simulink model "INS"  (R2018b)
settings: configuration reference "ins_config" (kept outside this file)
values from neighbouring files (symbols this model uses):
  INS_EXPORT = Simulink.Parameter(INS_EXPORT_VALUE)    [ins_model_init.m]
  INS_PARAM = Simulink.Parameter(INS_PARAM_VALUE)    [ins_model_init.m]
undefined symbols (not defined in the file or in its folder): DiscIntNeverNeededParam, INS_CONST, INS_EXPORT_VALUE
libraries: simulink x90, FMT_Model_Lib x31
(part 3 of 4)

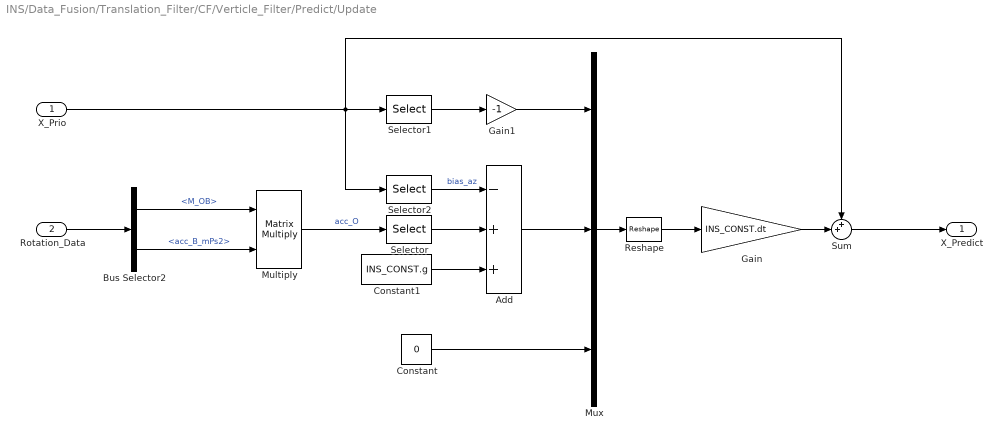
== system INS/Data_Fusion/Translation_Filter/CF/Verticle_Filter/Predict/Update ==
  X_Prio : Inport
  Rotation_Data : Inport  Port=2
  Add : Sum  Inputs=-++
  Bus Selector2 : BusSelector  OutputSignals=M_OB,acc_B_mPs2
  Constant : Constant  Value=0  OutDataTypeStr=single
  Constant1 : Constant  Value=INS_CONST.g  OutDataTypeStr=single
  Gain : Gain  Gain=INS_CONST.dt  OutDataTypeStr=Inherit: Same as input
  Gain1 : Gain  Gain=-1  OutDataTypeStr=Inherit: Same as input
  Multiply : Product  Multiplication=Matrix(*)
  Mux : Mux  Inputs=3
  Reshape : Reshape  OutputDimensionality=Customize  OutputDimensions=[3,1]
  Selector : Selector  InputPortWidth=3  IndexOptions=Index vector (dialog)  Indices=[3]  OutputSizes=1
  Selector1 : Selector  InputPortWidth=3  IndexOptions=Index vector (dialog)  Indices=[2]  OutputSizes=1
  Selector2 : Selector  InputPortWidth=3  IndexOptions=Index vector (dialog)  Indices=[3]  OutputSizes=1
  Sum : Sum  Inputs=++|
  X_Predict : Outport
  wires:
  Rotation_Data/1 -> Bus Selector2/1
  Bus Selector2/1 -> Multiply/1  "<M_OB>"
  Multiply/1 -> Selector/1  "acc_O"
  Bus Selector2/2 -> Multiply/2  "<acc_B_mPs2>"
  X_Prio/1 -> Selector2/1, Sum/1, Selector1/1
  Selector1/1 -> Gain1/1
  Constant/1 -> Mux/3
  Mux/1 -> Reshape/1
  Reshape/1 -> Gain/1
  Sum/1 -> X_Predict/1
  Add/1 -> Mux/2
  Constant1/1 -> Add/3
  Selector2/1 -> Add/1  "bias_az"
  Gain1/1 -> Mux/1
  Gain/1 -> Sum/2
  Selector/1 -> Add/2

== system INS/Data_Fusion/Translation_Filter/TF_Data_PreProcess/Sensor_Process/Sensor_Select/Horizontal_Sensor_Select ==
  Sensor_Status : Inport
  Bus Creator : BusCreator  Inputs=1
  Bus Selector : BusSelector  OutputSignals=GPS_Status.gps_vaid,GPS_Status.spd_valid,GPS_Status.pos_valid
  Compare To Zero2 : simulink/Logic and Bit Operations/Compare To Zero  relop=>  OutDataTypeStr=boolean
  Logical Operator : Logic  Inputs=3  AllPortsSameDT=off  OutDataTypeStr=boolean
  Min : MinMax
  horizon_select : Outport
  wires:
  Bus Selector/1 -> Logical Operator/1  "<gps_vaid>"
  Logical Operator/1 -> Min/1
  Min/1 -> Compare To Zero2/1
  Compare To Zero2/1 -> Bus Creator/1  "gps_enable"
  Sensor_Status/1 -> Bus Selector/1
  Bus Creator/1 -> horizon_select/1
  Bus Selector/2 -> Logical Operator/2  "<spd_valid>"
  Bus Selector/3 -> Logical Operator/3  "<pos_valid>"

== system INS/Data_Fusion/Translation_Filter/TF_Data_PreProcess/Sensor_Process/Sensor_Select/Vertical_Sensor_Select ==
  Sensor_Status : Inport
  Bus Creator : BusCreator  Inputs=2
  Bus Selector : BusSelector  OutputSignals=GPS_Status.gps_vaid,GPS_Status.spd_valid,GPS_Status.alt_valid
  Bus Selector2 : BusSelector  OutputSignals=Baro_Status.baro_valid
  Compare To Zero1 : simulink/Logic and Bit Operations/Compare To Zero  relop=>  OutDataTypeStr=boolean
  Compare To Zero4 : simulink/Logic and Bit Operations/Compare To Zero  relop=>  OutDataTypeStr=boolean
  Compare To Zero6 : simulink/Logic and Bit Operations/Compare To Zero  relop=>  OutDataTypeStr=boolean
  Data Type Conversion : DataTypeConversion  OutDataTypeStr=int8
  Data Type Conversion1 : DataTypeConversion  OutDataTypeStr=int8
  Logical Operator : Logic  Inputs=3  AllPortsSameDT=off  OutDataTypeStr=boolean
  Saturation : Saturate  UpperLimit=1  LowerLimit=0
  Saturation1 : Saturate  UpperLimit=1  LowerLimit=0
  Subtract : Sum  Inputs=-+
  vert_select : Outport
  wires:
  Data Type Conversion/1 -> Saturation/1
  Logical Operator/1 -> Data Type Conversion/1
  Saturation/1 -> Compare To Zero4/1, Subtract/1
  Bus Selector/2 -> Logical Operator/2  "<spd_valid>"
  Bus Selector2/1 -> Compare To Zero1/1  "<baro_valid>"
  Compare To Zero1/1 -> Data Type Conversion1/1
  Subtract/1 -> Saturation1/1
  Saturation1/1 -> Compare To Zero6/1
  Data Type Conversion1/1 -> Subtract/2
  Bus Selector/1 -> Logical Operator/1  "<gps_vaid>"
  Bus Selector/3 -> Logical Operator/3  "<alt_valid>"
  Compare To Zero4/1 -> Bus Creator/1  "gps_enable"
  Compare To Zero6/1 -> Bus Creator/2  "baro_enable"
  Sensor_Status/1 -> Bus Selector2/1, Bus Selector/1
  Bus Creator/1 -> vert_select/1

== system INS/Data_Fusion/Translation_Filter/TF_Data_PreProcess/Sensor_Process/TF_Sensor_Measures/Barometer_Meas ==
  Sensor_Data : Inport
  Bus Creator : BusCreator  Inputs=2
  Bus Selector1 : BusSelector  OutputSignals=Baro_Data.timestamp,Baro_Data.h_R_m
  Signal Copy1 : SignalConversion  OverrideOpt=off
  Signal Copy3 : SignalConversion  OverrideOpt=off
  Baro_Meas : Outport
  wires:
  Sensor_Data/1 -> Bus Selector1/1
  Bus Selector1/2 -> Signal Copy1/1  "<h_R_m>"
  Bus Creator/1 -> Baro_Meas/1
  Bus Selector1/1 -> Signal Copy3/1  "<timestamp>"
  Signal Copy3/1 -> Bus Creator/1  "timestamp_ms"
  Signal Copy1/1 -> Bus Creator/2  "h_R_m"

== system INS/Data_Fusion/Translation_Filter/TF_Data_PreProcess/Sensor_Process/TF_Sensor_Measures/GPS_Meas ==
  Sensor_Data : Inport
  Bus Creator : BusCreator  Inputs=12
  Bus Selector : BusSelector  OutputSignals=GPS_Data.dx_dlat,GPS_Data.dy_dlon,GPS_Data.dz_dh,GPS_Data.lat_rad,GPS_Data.lon_rad,GPS_Data.height_m,GPS_Data.vn_mPs,GPS_Data.ve_mPs,GPS_Data.vd_mPs,GPS_Data.timestamp_ms,GPS_Data.spd_quality,GPS_Data.pos_quality
  Signal Copy{,1..11} (12 alike) : SignalConversion  OverrideOpt=off
  GPS_Meas : Outport
  wires:
  Bus Selector/11 -> Signal Copy10/1  "<spd_quality>"
  Signal Copy9/1 -> Bus Creator/10  "timestamp_ms"
  Signal Copy8/1 -> Bus Creator/9  "vd_mPs"
  Signal Copy7/1 -> Bus Creator/8  "ve_mPs"
  Signal Copy6/1 -> Bus Creator/7  "vn_mPs"
  Signal Copy5/1 -> Bus Creator/6  "h_m"
  Signal Copy4/1 -> Bus Creator/5  "lon_rad"
  Signal Copy3/1 -> Bus Creator/4  "lat_rad"
  Signal Copy2/1 -> Bus Creator/3  "dz_dh"
  Signal Copy1/1 -> Bus Creator/2  "dy_dlon"
  Signal Copy/1 -> Bus Creator/1  "dx_dlat"
  Bus Selector/10 -> Signal Copy9/1  "<timestamp_ms>"
  Bus Selector/9 -> Signal Copy8/1  "<vd_mPs>"
  Bus Selector/8 -> Signal Copy7/1  "<ve_mPs>"
  Bus Selector/7 -> Signal Copy6/1  "<vn_mPs>"
  Bus Selector/6 -> Signal Copy5/1  "<height_m>"
  Bus Selector/5 -> Signal Copy4/1  "<lon_rad>"
  Bus Selector/4 -> Signal Copy3/1  "<lat_rad>"
  Bus Selector/3 -> Signal Copy2/1  "<dz_dh>"
  Bus Selector/2 -> Signal Copy1/1  "<dy_dlon>"
  Bus Selector/1 -> Signal Copy/1  "<dx_dlat>"
  Bus Creator/1 -> GPS_Meas/1
  Sensor_Data/1 -> Bus Selector/1
  Bus Selector/12 -> Signal Copy11/1  "<pos_quality>"
  Signal Copy10/1 -> Bus Creator/11  "spd_quality"
  Signal Copy11/1 -> Bus Creator/12  "pos_quality"

== system INS/Data_Fusion/Translation_Filter/TF_Data_PreProcess/Sensor_Process/TF_Sensor_Status/Barometer_Status ==
  Sensor_Data : Inport
  Bus Creator : BusCreator  Inputs=1
  Bus Selector : BusSelector  OutputSignals=Baro_Data.baro_valid
  Signal Copy : SignalConversion  OverrideOpt=off
  Baro_Status : Outport
  wires:
  Bus Selector/1 -> Signal Copy/1  "<baro_valid>"
  Bus Creator/1 -> Baro_Status/1
  Sensor_Data/1 -> Bus Selector/1
  Signal Copy/1 -> Bus Creator/1  "baro_valid"

== system INS/Data_Fusion/Translation_Filter/TF_Data_PreProcess/Sensor_Process/TF_Sensor_Status/GPS_Status ==
  Sensor_Data : Inport
  Bus Creator : BusCreator  Inputs=4
  Bus Selector : BusSelector  OutputSignals=GPS_Data.GPS_valid,GPS_Data.spd_quality,GPS_Data.pos_quality,GPS_Data.alt_quality
  Relay : Relay  OnSwitchValue=0.7  OffSwitchValue=0.3
  Relay1 : Relay  OnSwitchValue=0.7  OffSwitchValue=0.3
  Relay2 : Relay  OnSwitchValue=0.7  OffSwitchValue=0.3
  Signal Copy : SignalConversion  OverrideOpt=off
  GPS_Status : Outport
  wires:
  Bus Creator/1 -> GPS_Status/1
  Relay1/1 -> Bus Creator/3  "pos_valid"
  Relay/1 -> Bus Creator/2  "spd_valid"
  Signal Copy/1 -> Bus Creator/1  "gps_vaid"
  Bus Selector/3 -> Relay1/1  "<pos_quality>"
  Bus Selector/2 -> Relay/1  "<spd_quality>"
  Bus Selector/1 -> Signal Copy/1  "<GPS_valid>"
  Sensor_Data/1 -> Bus Selector/1
  Bus Selector/4 -> Relay2/1  "<alt_quality>"
  Relay2/1 -> Bus Creator/4  "alt_valid"

== system INS/Data_Fusion/Translation_Filter/TF_Data_PreProcess/Transfer_Filter_Control/Position_Reference/Bus_Constructor ==
  WGS84_pos_ref : Inport
  WGS84_dpos_ref : Inport  Port=2
  WGS84_hgt_ref : Inport  Port=3
  WGS84_dhgt_ref : Inport  Port=4
  Bus Creator : BusCreator  Inputs=2
  Bus Creator1 : BusCreator  Inputs=3
  Bus Creator2 : BusCreator  Inputs=3
  Demux : Demux  Outputs=2
  Demux1 : Demux  Outputs=2
  WGS84_Ref : Outport
  wires:
  Bus Creator/1 -> WGS84_Ref/1
  Demux/1 -> Bus Creator1/1  "dx_dlat_0"
  Demux1/1 -> Bus Creator2/1  "lat_0_rad"
  Demux/2 -> Bus Creator1/2  "dy_dlon_0"
  Demux1/2 -> Bus Creator2/2  "lon_0_rad"
  Bus Creator2/1 -> Bus Creator/2  "WGS84_pos_ref"
  WGS84_dhgt_ref/1 -> Bus Creator1/3  "dz_dh_0"
  WGS84_hgt_ref/1 -> Bus Creator2/3  "h_0_m"
  Bus Creator1/1 -> Bus Creator/1  "WGS84_derivatives_ref"
  WGS84_dpos_ref/1 -> Demux/1
  WGS84_pos_ref/1 -> Demux1/1

== system INS/Data_Fusion/Translation_Filter/TF_Data_PreProcess/Transfer_Filter_Control/Position_Reference/Bus_Select ==
  Sensor_Meas : Inport
  Bus Selector1 : BusSelector  OutputSignals=GPS_Meas.dx_dlat,GPS_Meas.dy_dlon,GPS_Meas.dz_dh,GPS_Meas.lat_rad,GPS_Meas.lon_rad,GPS_Meas.h_m
  Mux : Mux  Inputs=3
  Mux1 : Mux  Inputs=3
  WGS84_derivatives : Outport
  WGS84_position : Outport  Port=2
  wires:
  Mux1/1 -> WGS84_position/1
  Sensor_Meas/1 -> Bus Selector1/1
  Mux/1 -> WGS84_derivatives/1
  Bus Selector1/6 -> Mux1/3  "<h_m>"
  Bus Selector1/5 -> Mux1/2  "<lon_rad>"
  Bus Selector1/4 -> Mux1/1  "<lat_rad>"
  Bus Selector1/3 -> Mux/3  "<dz_dh>"
  Bus Selector1/2 -> Mux/2  "<dy_dlon>"
  Bus Selector1/1 -> Mux/1  "<dx_dlat>"

== system INS/Data_Fusion/Translation_Filter/TF_Data_PreProcess/Transfer_Filter_Control/Position_Reference/Height_Ref ==
  Translation_Data : Inport
  Sensor_Valid : Inport  Port=2
  WGS84_derivatives : Inport  Port=3
  WGS84_position : Inport  Port=4
  Bus Selector1 : BusSelector  OutputSignals=h_R_m
  Bus Selector2 : BusSelector  OutputSignals=altitude_valid
  Delay : Delay  DelayLength=1
  Delay1 : Delay  DelayLength=1
  Detect Rise Positive3 : simulink/Logic and Bit Operations/Detect Rise Positive  vinit=0  OutDataTypeStr=boolean
  Selector : Selector  InputPortWidth=3  IndexOptions=Index vector (dialog)  Indices=3  OutputSizes=1
  Selector1 : Selector  InputPortWidth=3  IndexOptions=Index vector (dialog)  Indices=3  OutputSizes=1
  Sum : Sum  Inputs=|+-
  Switch1 : Switch  Criteria=u2 > Threshold
  Switch4 : Switch  Criteria=u2 > Threshold
  WGS84_hgt_ref : Outport
  WGS84_dhgt_ref : Outport  Port=2
  wires:
  Delay1/1 -> Switch4/3
  Switch4/1 -> WGS84_hgt_ref/1, Delay1/1
  Detect Rise Positive3/1 -> Switch1/2, Switch4/2
  Bus Selector2/1 -> Detect Rise Positive3/1  "<altitude_valid>"
  WGS84_derivatives/1 -> Selector/1
  Switch1/1 -> WGS84_dhgt_ref/1, Delay/1
  Delay/1 -> Switch1/3
  Sensor_Valid/1 -> Bus Selector2/1
  Translation_Data/1 -> Bus Selector1/1
  Sum/1 -> Switch4/1
  WGS84_position/1 -> Selector1/1
  Selector/1 -> Switch1/1
  Selector1/1 -> Sum/1
  Bus Selector1/1 -> Sum/2  "<h_R_m>"

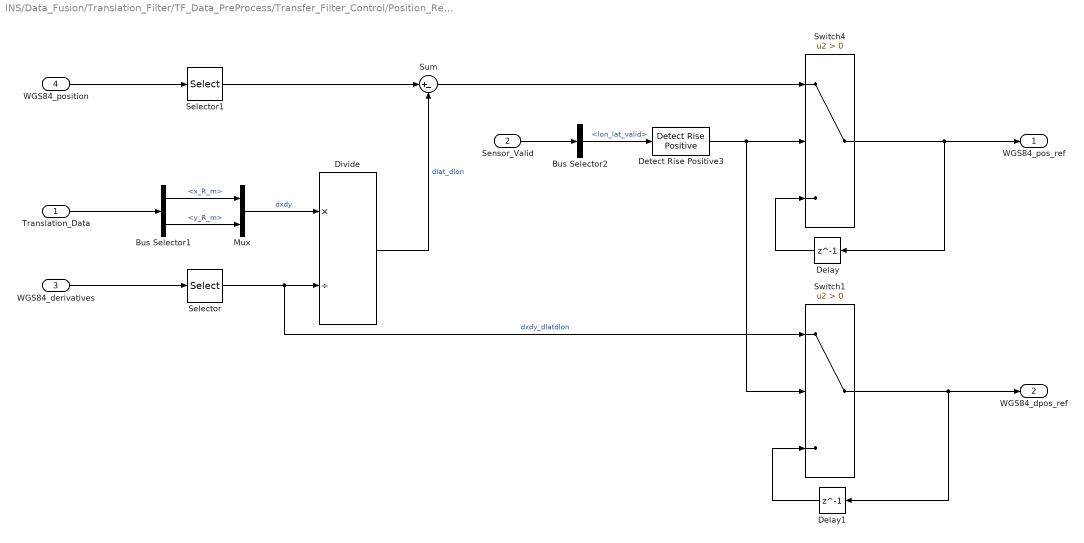
== system INS/Data_Fusion/Translation_Filter/TF_Data_PreProcess/Transfer_Filter_Control/Position_Reference/Position_Ref ==
  Translation_Data : Inport
  Sensor_Valid : Inport  Port=2
  WGS84_derivatives : Inport  Port=3
  WGS84_position : Inport  Port=4
  Bus Selector1 : BusSelector  OutputSignals=x_R_m,y_R_m
  Bus Selector2 : BusSelector  OutputSignals=lon_lat_valid
  Delay : Delay  DelayLength=1
  Delay1 : Delay  DelayLength=1
  Detect Rise Positive3 : simulink/Logic and Bit Operations/Detect Rise Positive  vinit=0  OutDataTypeStr=boolean
  Divide : Product  Inputs=*/
  Mux : Mux  Inputs=2
  Selector : Selector  InputPortWidth=3  IndexOptions=Index vector (dialog)  Indices=[1 2]  OutputSizes=1
  Selector1 : Selector  InputPortWidth=3  IndexOptions=Index vector (dialog)  Indices=[1 2]  OutputSizes=1
  Sum : Sum  Inputs=|+-
  Switch1 : Switch  Criteria=u2 > Threshold
  Switch4 : Switch  Criteria=u2 > Threshold
  WGS84_pos_ref : Outport
  WGS84_dpos_ref : Outport  Port=2
  wires:
  Delay/1 -> Switch4/3
  Bus Selector1/1 -> Mux/1  "<x_R_m>"
  Switch4/1 -> WGS84_pos_ref/1, Delay/1
  Mux/1 -> Divide/1  "dxdy"
  Detect Rise Positive3/1 -> Switch1/2, Switch4/2
  Bus Selector2/1 -> Detect Rise Positive3/1  "<lon_lat_valid>"
  WGS84_derivatives/1 -> Selector/1
  Switch1/1 -> Delay1/1, WGS84_dpos_ref/1
  Delay1/1 -> Switch1/3
  Sensor_Valid/1 -> Bus Selector2/1
  Translation_Data/1 -> Bus Selector1/1
  Sum/1 -> Switch4/1
  Bus Selector1/2 -> Mux/2  "<y_R_m>"
  Divide/1 -> Sum/2  "dlat_dlon"
  WGS84_position/1 -> Selector1/1
  Selector/1 -> Switch1/1, Divide/2  "dxdy_dlatdlon"
  Selector1/1 -> Sum/1

== system INS/Data_Fusion/Translation_Filter/TF_Data_PreProcess/Transfer_Filter_Control/Sensor_Valid/Horizon_Sensor_Valid ==
  Sensor_Enable : Inport
  Bus Selector1 : BusSelector  OutputSignals=horizon_select.gps_enable
  Signal Copy : SignalConversion  OverrideOpt=off
  valid_hold : Subsystem  mask{time_out=1000}
      mask prompts: time_out "timeout in ms"
  valid_hold1 : Subsystem  mask{time_out=1000}
      mask prompts: time_out "timeout in ms"
  lon_lat_valid : Outport
  xy_R_valid : Outport  Port=2
  wires:
  Sensor_Enable/1 -> Bus Selector1/1
  Bus Selector1/1 -> Signal Copy/1  "<gps_enable>"
  Signal Copy/1 -> valid_hold1/1(u), valid_hold/1(u)
  valid_hold/1(y) -> lon_lat_valid/1
  valid_hold1/1(y) -> xy_R_valid/1

== system INS/Data_Fusion/Translation_Filter/TF_Data_PreProcess/Transfer_Filter_Control/Sensor_Valid/Vertical_Sensor_Valid ==
  Sensor_Enable : Inport
  Bus Selector1 : BusSelector  OutputSignals=vert_select.gps_enable,vert_select.baro_enable
  Logical Operator : Logic  Operator=OR  AllPortsSameDT=off  OutDataTypeStr=boolean
  Signal Copy : SignalConversion  OverrideOpt=off
  valid_hold : Subsystem  mask{time_out=1000}
      mask prompts: time_out "timeout in ms"
  valid_hold1 : Subsystem  mask{time_out=1000}
      mask prompts: time_out "timeout in ms"
  altitude_valid : Outport
  h_R_valid : Outport  Port=2
  wires:
  Sensor_Enable/1 -> Bus Selector1/1
  Bus Selector1/1 -> Signal Copy/1  "<gps_enable>"
  Signal Copy/1 -> valid_hold/1(u), Logical Operator/1
  Bus Selector1/2 -> Logical Operator/2  "<baro_enable>"
  Logical Operator/1 -> valid_hold1/1(u)
  valid_hold/1(y) -> altitude_valid/1
  valid_hold1/1(y) -> h_R_valid/1

== system INS/Sensor_PreProcess/MAG_PreProcess/Mag_Data_Process/Mag_Quality_Estimate/Mag_Quality/Inclination_Quality_Estimate ==
  nominal_inc_deg : Inport
  mag_normalized_O : Inport  Port=2
  Abs1 : Abs
  Constant2 : Constant  OutDataTypeStr=Inherit: Inherit via back propagation
  Gain1 : Gain  Gain=pi/180
  Saturation : Saturate  UpperLimit=1  LowerLimit=0
  Selector : Selector  InputPortWidth=3  IndexOptions=Index vector (dialog)  Indices=[1 2]  OutputSizes=1
  Selector1 : Selector  InputPortWidth=3  IndexOptions=Index vector (dialog)  Indices=3  OutputSizes=1
  Subtract : Sum  Inputs=+-
  Sum3 : Sum  Inputs=+-|
  Trigonometric Function : Trigonometry  Operator=atan2
  Vector Modulus : FMT_Model_Lib/Math/Vector Modulus
      settings: SourceProductName=FMT Toolbox
  gain : Gain  Gain=2
  inclination_quality : Outport
  wires:
  mag_normalized_O/1 -> Selector1/1, Selector/1
  Trigonometric Function/1 -> Subtract/2
  Vector Modulus/1 -> Trigonometric Function/2
  Abs1/1 -> gain/1
  gain/1 -> Sum3/2
  Gain1/1 -> Subtract/1
  Subtract/1 -> Abs1/1
  Constant2/1 -> Sum3/1
  nominal_inc_deg/1 -> Gain1/1
  Sum3/1 -> Saturation/1
  Selector/1 -> Vector Modulus/1
  Selector1/1 -> Trigonometric Function/1
  Saturation/1 -> inclination_quality/1

== system INS/Sensor_PreProcess/MAG_PreProcess/Mag_Data_Process/Mag_Quality_Estimate/Mag_Quality/Intensity_Quality_Estimate ==
  mag_normalized_O : Inport
  Abs : Abs
  Constant1 : Constant  OutDataTypeStr=Inherit: Inherit via back propagation
  Nominal_Magnitude : Constant  OutDataTypeStr=Inherit: Inherit via back propagation
  Saturation : Saturate  UpperLimit=1  LowerLimit=0
  Subtract : Sum  Inputs=+-
  Sum : Sum  Inputs=+-|
  Vector Modulus : FMT_Model_Lib/Math/Vector Modulus
      settings: SourceProductName=FMT Toolbox
  gain : Gain
  intensity_quality : Outport
  wires:
  Constant1/1 -> Sum/1
  Vector Modulus/1 -> Subtract/2
  Subtract/1 -> Abs/1
  Sum/1 -> Saturation/1
  Nominal_Magnitude/1 -> Subtract/1
  Saturation/1 -> intensity_quality/1
  Abs/1 -> gain/1  "magnitude_error"
  gain/1 -> Sum/2
  mag_normalized_O/1 -> Vector Modulus/1

== system INS/Data_Fusion/Rotation_Filter/AHRS/Correct/Attitude_Correction/Attitude_Correct/Acc_Correct ==
  acc_meas_valid : Inport
  acc_meas_O_mPs2 : Inport  Port=2
  acc_est_O_mPs2 : Inport  Port=3
  Heading_Correct : Subsystem
  Sum : Sum  Inputs=|++
  Verticle_Correct : Subsystem
  att_correct : Outport
  wires:
  acc_meas_valid/1 -> Heading_Correct/3(acc_meas_valid)
  Verticle_Correct/1(vert_correct) -> Sum/1  "vert_correct"
  Heading_Correct/1(heading_correct) -> Sum/2  "heading_correct"
  acc_meas_O_mPs2/1 -> Verticle_Correct/2(acc_meas_O_mPs2), Heading_Correct/2(acc_meas_O_mPs2)
  acc_est_O_mPs2/1 -> Verticle_Correct/1(acc_est_O_mPs2), Heading_Correct/1(acc_est_O_mPs2)
  Sum/1 -> att_correct/1

== system INS/Data_Fusion/Rotation_Filter/AHRS/Correct/Attitude_Correction/Attitude_Correct/Acc_Estimator ==
  Sensor_Data : Inport
  Rotation_Data : Inport  Port=2
  Estimate_Acc : Subsystem
  Measure_Acc : Subsystem
  Multiply : Product  OutDataTypeStr=single
  Sum2 : Sum  Inputs=++|
  gravity : Constant  Value=[0;0;-INS_CONST.g]  VectorParams1D=off  OutDataTypeStr=single
  acc_meas_valid : Outport
  acc_meas_O_mPs2 : Outport  Port=2
  acc_est_O_mPs2 : Outport  Port=3
  wires:
  Measure_Acc/1(gps_meas_valid) -> Estimate_Acc/1(gps_meas_valid), acc_meas_valid/1, Multiply/1
  Sum2/1 -> acc_meas_O_mPs2/1
  Sensor_Data/1 -> Estimate_Acc/2(Sensor_Data), Measure_Acc/1(Sensor_Data)
  gravity/1 -> Sum2/1
  Multiply/1 -> Sum2/2
  Measure_Acc/2(gps_meas_acc) -> Multiply/2
  Rotation_Data/1 -> Estimate_Acc/3(Rotation_Data)
  Estimate_Acc/1(acc_est_O_mPs2) -> acc_est_O_mPs2/1

== system INS/Data_Fusion/Rotation_Filter/AHRS/Correct/Attitude_Correction/Mag_Correct/Subsystem ==
  M_OB : Inport
  mag_B : Inport  Port=2
  Rotation_Data : Inport  Port=3
  Add : Sum
  Atan2 : Trigonometry  Operator=atan2
  Bus Selector : BusSelector  OutputSignals=psi_rad
  Demux : Demux  Outputs=3
  Gain : Gain  Gain=-1
  MX Product1 : Product  Multiplication=Matrix(*)  RndMeth=Simplest
  Terminator : Terminator
  Terminator1 : Terminator
  wires:
  Demux/3 -> Terminator1/1
  Atan2/1 -> Add/1
  Demux/1 -> Atan2/2
  MX Product1/1 -> Demux/1  "my_O"
  Gain/1 -> Atan2/1
  Add/1 -> Terminator/1  "mag_heading"
  Rotation_Data/1 -> Bus Selector/1
  Bus Selector/1 -> Add/2  "<psi_rad>"
  Demux/2 -> Gain/1
  mag_B/1 -> MX Product1/2
  M_OB/1 -> MX Product1/1

== system INS/Data_Fusion/Translation_Filter/CF/Bus_Constructor/Bus_Select/WGS84_Position/WGS84_Position ==
  xyh_R_m : Inport
  TF_Data : Inport  Port=2
  Bus Selector : BusSelector  OutputSignals=TF_Control.WGS84_Ref.WGS84_derivatives_ref.dx_dlat_0,TF_Control.WGS84_Ref.WGS84_derivatives_ref.dy_dlon_0
  Bus Selector1 : BusSelector  OutputSignals=TF_Control.WGS84_Ref.WGS84_pos_ref.lat_0_rad,TF_Control.WGS84_Ref.WGS84_pos_ref.lon_0_rad,TF_Control.WGS84_Ref.WGS84_pos_ref.h_0_m
  Data Type Conversion : DataTypeConversion  OutDataTypeStr=double
  Data Type Conversion1 : DataTypeConversion  OutDataTypeStr=double
  Mux : Mux  Inputs=2
  Mux1 : Mux  Inputs=2
  Mux2 : Mux  Inputs=3
  Selector : Selector  InputPortWidth=3  IndexOptions=Index vector (dialog)  Indices=[1 2]  OutputSizes=1
  Selector1 : Selector  InputPortWidth=3  IndexOptions=Index vector (dialog)  Indices=[3]  OutputSizes=1
  Sum : Sum  Inputs=|++
  safe_divide : Subsystem
  WGS84_pos : Outport
  wires:
  Selector/1 -> Data Type Conversion/1
  Mux/1 -> safe_divide/2(u2)
  Selector1/1 -> Data Type Conversion1/1
  Data Type Conversion1/1 -> Mux1/2
  Bus Selector/1 -> Mux/1  "<dx_dlat_0>"
  xyh_R_m/1 -> Selector1/1, Selector/1
  Bus Selector/2 -> Mux/2  "<dy_dlon_0>"
  safe_divide/1(y) -> Mux1/1
  Data Type Conversion/1 -> safe_divide/1(u1)
  Mux1/1 -> Sum/1
  Bus Selector1/2 -> Mux2/2  "<lon_0_rad>"
  TF_Data/1 -> Bus Selector1/1, Bus Selector/1
  Bus Selector1/3 -> Mux2/3  "<h_0_m>"
  Bus Selector1/1 -> Mux2/1  "<lat_0_rad>"
  Mux2/1 -> Sum/2
  Sum/1 -> WGS84_pos/1

== system INS/Data_Fusion/Translation_Filter/CF/Horizontal_Filter/Correct/GPS_Correct/Error_Integrate ==
  error : Inport
  update : Inport  Port=2
  Gain3 : Gain  Gain=INS_CONST.dt  OutDataTypeStr=Inherit: Same as input
  Memory : Memory
  Switch : Switch  Criteria=u2 > Threshold
  corr : Outport
  wires:
  update/1 -> Switch/2
  Switch/1 -> Memory/1, Gain3/1
  error/1 -> Switch/1
  Memory/1 -> Switch/3
  Gain3/1 -> corr/1

== system INS/Data_Fusion/Translation_Filter/CF/Horizontal_Filter/Correct/GPS_Correct/Error_Scaling ==
  err_in : Inport
  Demux : Demux  Outputs=2
  Gain : Gain  Gain=INS_PARAM.GPS_VEL_CORR_GAIN  OutDataTypeStr=single
  Gain1 : Gain  Commented=on  Gain=1.5  OutDataTypeStr=single
  Gain2 : Gain  Gain=-INS_PARAM.GPS_BIAS_A_CORR_GAIN  OutDataTypeStr=single
  Gain3 : Gain  Gain=INS_PARAM.GPS_POS_CORR_GAIN  OutDataTypeStr=single
  Mux : Mux  Inputs=3
  Reshape : Reshape  OutputDimensionality=Customize  OutputDimensions=[6,1]
  err_out : Outport
  wires:
  err_in/1 -> Demux/1
  Demux/1 -> Gain3/1
  Demux/2 -> Gain2/1, Gain/1
  Gain2/1 -> Mux/3
  Mux/1 -> Reshape/1
  Gain3/1 -> Mux/1
  Gain/1 -> Mux/2
  Reshape/1 -> err_out/1

== system INS/Data_Fusion/Translation_Filter/CF/Horizontal_Filter/Correct/GPS_Correct/Estimate_State ==
  X : Inport
  reset : Inport  Port=2
  Mux : Mux
  Reshape : Reshape  OutputDimensionality=Customize  OutputDimensions=[4,1]
  Selector : Selector  InputPortWidth=6  IndexOptions=Index vector (dialog)  Indices=[1]  OutputSizes=1
  Selector1 : Selector  InputPortWidth=6  IndexOptions=Index vector (dialog)  Indices=[2]  OutputSizes=1
  Selector2 : Selector  InputPortWidth=6  IndexOptions=Index vector (dialog)  Indices=[3]  OutputSizes=1
  Selector3 : Selector  InputPortWidth=6  IndexOptions=Index vector (dialog)  Indices=[4]  OutputSizes=1
  vn_delay : Delay  DelayLength=INS_PARAM.GPS_VEL_DELAY/INS_EXPORT.period  InitialConditionSource=Input port  ExternalReset=Rising
      settings: InputPortMap=u0,r5,p4
  vn_delay1 : Delay  DelayLength=INS_PARAM.GPS_VEL_DELAY/INS_EXPORT.period  InitialConditionSource=Input port  ExternalReset=Rising
      settings: InputPortMap=u0,r5,p4
  x_delay : Delay  DelayLength=INS_PARAM.GPS_POS_DELAY/INS_EXPORT.period  InitialConditionSource=Input port  ExternalReset=Rising
      settings: InputPortMap=u0,r5,p4
  x_delay1 : Delay  DelayLength=INS_PARAM.GPS_POS_DELAY/INS_EXPORT.period  InitialConditionSource=Input port  ExternalReset=Rising
      settings: InputPortMap=u0,r5,p4
  HX : Outport
  wires:
  Mux/1 -> Reshape/1
  Reshape/1 -> HX/1
  reset/1 -> vn_delay1/2, x_delay/2, x_delay1/2, vn_delay/2
  x_delay1/1 -> Mux/2
  vn_delay/1 -> Mux/3
  vn_delay1/1 -> Mux/4
  x_delay/1 -> Mux/1
  Selector/1 -> x_delay/3, x_delay/1
  X/1 -> Selector3/1, Selector2/1, Selector1/1, Selector/1
  Selector1/1 -> x_delay1/3, x_delay1/1
  Selector2/1 -> vn_delay/3, vn_delay/1
  Selector3/1 -> vn_delay1/3, vn_delay1/1

== system INS/Data_Fusion/Translation_Filter/CF/Horizontal_Filter/Correct/GPS_Correct/Measurement ==
  X : Inport
  TF_Data : Inport  Port=2
  Bias_Estimation : Subsystem
  Bus Selector : BusSelector  OutputSignals=Sensor_Meas.GPS_Meas.lat_rad,Sensor_Meas.GPS_Meas.lon_rad,TF_Control.WGS84_Ref.WGS84_pos_ref.lat_0_rad,TF_Control.WGS84_Ref.WGS84_pos_ref.lon_0_rad,TF_Control.WGS84_Ref.WGS84_derivatives_ref.dx_dlat_0,TF_Control.WGS84_Ref.WGS84_derivatives_ref.dy_dlon_0
  Bus Selector1 : BusSelector  OutputSignals=Sensor_Meas.GPS_Meas.vn_mPs,Sensor_Meas.GPS_Meas.ve_mPs
  Data Type Conversion : DataTypeConversion  OutDataTypeStr=single
  Multiply : Product
  Mux{,1..4} (5 alike) : Mux  Inputs=2
  Reshape3 : Reshape  OutputDimensionality=Customize  OutputDimensions=[4,1]
  Sum : Sum  Inputs=|+-
  Z : Outport
  bias_update : Outport  Port=2
  wires:
  X/1 -> Bias_Estimation/2(X)
  Data Type Conversion/1 -> Bias_Estimation/3(xy_meas_m)
  Bias_Estimation/2(xy_O_m) -> Mux3/1
  Bus Selector1/2 -> Mux4/2  "<ve_mPs>"
  Bus Selector1/1 -> Mux4/1  "<vn_mPs>"
  Multiply/1 -> Data Type Conversion/1  "xy"
  Mux2/1 -> Multiply/2
  Sum/1 -> Multiply/1
  Bus Selector/6 -> Mux2/2  "<dy_dlon_0>"
  Bus Selector/5 -> Mux2/1  "<dx_dlat_0>"
  Mux1/1 -> Sum/2
  Mux/1 -> Sum/1
  Bus Selector/4 -> Mux1/2  "<lon_0_rad>"
  Bus Selector/3 -> Mux1/1  "<lat_0_rad>"
  Bus Selector/2 -> Mux/2  "<lon_rad>"
  Bus Selector/1 -> Mux/1  "<lat_rad>"
  TF_Data/1 -> Bus Selector/1, Bus Selector1/1, Bias_Estimation/1(TF_Data)
  Bias_Estimation/1(bias_update) -> bias_update/1
  Mux3/1 -> Reshape3/1
  Reshape3/1 -> Z/1
  Mux4/1 -> Mux3/2

== system INS/Data_Fusion/Translation_Filter/CF/Horizontal_Filter/Predict/Propagate/States_Init ==
  TF_Data : Inport
  Constant : Constant  Value=[0;0]  VectorParams1D=off  OutDataTypeStr=single
  Mux : Mux  Inputs=3
  Pos_Init : Subsystem
  Vel_Init : Subsystem
  X_0 : Outport
  wires:
  TF_Data/1 -> Pos_Init/1(TF_Data), Vel_Init/1(TF_Data)
  Constant/1 -> Mux/3  "ba_xy_0"
  Mux/1 -> X_0/1
  Vel_Init/1(vel_NE_0) -> Mux/2
  Pos_Init/1(XY_0) -> Mux/1

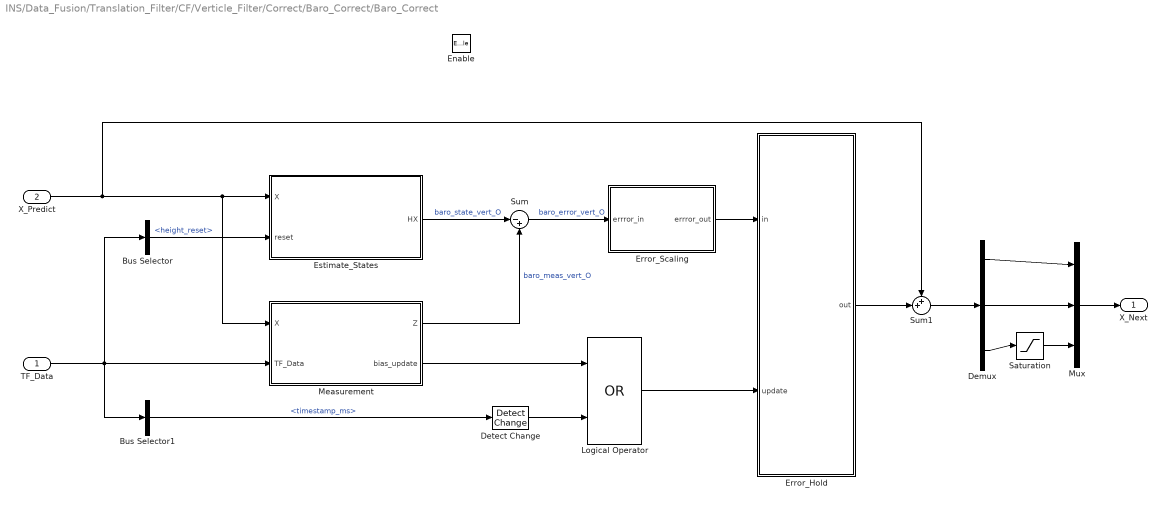
== system INS/Data_Fusion/Translation_Filter/CF/Verticle_Filter/Correct/Baro_Correct/Baro_Correct ==
  TF_Data : Inport
  X_Predict : Inport  Port=2
  Enable : EnablePort  StatesWhenEnabling=reset
  Bus Selector : BusSelector  OutputSignals=TF_Control.height_reset
  Bus Selector1 : BusSelector  OutputSignals=Sensor_Meas.Baro_Meas.timestamp_ms
  Demux : Demux  Outputs=3
  Detect Change : simulink/Logic and Bit Operations/Detect Change  vinit=0  OutDataTypeStr=boolean
  Error_Hold : Subsystem
  Error_Scaling : Subsystem  mask{w=1.2}
      mask prompts: w "omega"
  Estimate_States : Subsystem
  Logical Operator : Logic  Operator=OR  AllPortsSameDT=off  OutDataTypeStr=boolean
  Measurement : Subsystem
  Mux : Mux  Inputs=3
  Saturation : Saturate
  Sum : Sum  Inputs=|-+
  Sum1 : Sum  Inputs=++|
  X_Next : Outport
  wires:
  Estimate_States/1(HX) -> Sum/1  "baro_state_vert_O"
  Measurement/1(Z) -> Sum/2  "baro_meas_vert_O"
  TF_Data/1 -> Bus Selector/1, Measurement/2(TF_Data), Bus Selector1/1
  Sum/1 -> Error_Scaling/1(errror_in)  "baro_error_vert_O"
  Bus Selector1/1 -> Detect Change/1  "<timestamp_ms>"
  Error_Hold/1(out) -> Sum1/2
  Sum1/1 -> Demux/1
  X_Predict/1 -> Measurement/1(X), Estimate_States/1(X), Sum1/1
  Bus Selector/1 -> Estimate_States/2(reset)  "<height_reset>"
  Logical Operator/1 -> Error_Hold/2(update)
  Detect Change/1 -> Logical Operator/2
  Measurement/2(bias_update) -> Logical Operator/1
  Error_Scaling/1(errror_out) -> Error_Hold/1(in)
  Demux/3 -> Saturation/1
  Mux/1 -> X_Next/1
  Saturation/1 -> Mux/3
  Demux/2 -> Mux/2
  Demux/1 -> Mux/1

== system INS/Data_Fusion/Translation_Filter/CF/Verticle_Filter/Correct/GPS_Correct/GPS_Correct ==
  TF_Data : Inport
  X_Predict : Inport  Port=2
  Enable : EnablePort  StatesWhenEnabling=reset
  Bus Selector : BusSelector  OutputSignals=TF_Control.height_reset
  Bus Selector1 : BusSelector  OutputSignals=Sensor_Meas.Baro_Meas.timestamp_ms
  Detect Change : simulink/Logic and Bit Operations/Detect Change  vinit=0  OutDataTypeStr=boolean
  Error_Hold : Subsystem
  Error_Scaling : Subsystem
  Estimate_State : Subsystem
  Logical Operator : Logic  Operator=OR  AllPortsSameDT=off  OutDataTypeStr=boolean
  Measurement : Subsystem
  Sum : Sum  Inputs=|-+
  Sum1 : Sum  Inputs=++|
  X_Next : Outport
  wires:
  Estimate_State/1(HX) -> Sum/1  "gps_state_vert_O"
  Measurement/1(Z) -> Sum/2  "gps_meas_vert_O"
  TF_Data/1 -> Bus Selector/1, Measurement/2(TF_Data), Bus Selector1/1
  Sum/1 -> Error_Scaling/1(error_in)  "gps_error_vert_O"
  Bus Selector1/1 -> Detect Change/1  "<timestamp_ms>"
  Error_Hold/1(out) -> Sum1/2
  Sum1/1 -> X_Next/1
  X_Predict/1 -> Measurement/1(X), Estimate_State/1(X), Sum1/1
  Bus Selector/1 -> Estimate_State/2(reset)  "<height_reset>"
  Logical Operator/1 -> Error_Hold/2(update)
  Detect Change/1 -> Logical Operator/2
  Measurement/2(bias_update) -> Logical Operator/1
  Error_Scaling/1(error_out) -> Error_Hold/1(in)

== system INS/Data_Fusion/Translation_Filter/CF/Verticle_Filter/Predict/Propagate/States_Init ==
  TF_Data : Inport
  Baro_Height_Init : Subsystem
  Constant : Constant  Value=0  OutDataTypeStr=single
  GPS_Height_Init : Subsystem
  Merge : Merge
  Merge1 : Merge
  Mux : Mux  Inputs=3
  X_0 : Outport
  wires:
  Constant/1 -> Mux/3  "ba_z_0"
  Mux/1 -> X_0/1
  TF_Data/1 -> Baro_Height_Init/1(TF_Data), GPS_Height_Init/1(TF_Data)
  Merge/1 -> Mux/1  "h_0"
  GPS_Height_Init/1(h_0) -> Merge/1
  Merge1/1 -> Mux/2  "vel_D_0"
  GPS_Height_Init/2(vel_D) -> Merge1/1
  Baro_Height_Init/1(h_0) -> Merge/2
  Baro_Height_Init/2(vel_D) -> Merge1/2

== system INS/Data_Fusion/Translation_Filter/TF_Data_PreProcess/Transfer_Filter_Control/Sensor_Valid/Horizon_Sensor_Valid/valid_hold ==
  u : Inport
  Compare To Constant : simulink/Logic and Bit Operations/Compare To Constant  relop=>=  const=time_out  OutDataTypeStr=boolean
  Compare To Constant1 : simulink/Logic and Bit Operations/Compare To Constant  relop=>  const=0  OutDataTypeStr=boolean
  Compare To Constant2 : simulink/Logic and Bit Operations/Compare To Constant  relop=>  const=0  OutDataTypeStr=boolean
  Constant : Constant  Value=INS_EXPORT.period  OutDataTypeStr=Inherit: Inherit via back propagation
  Delay : Delay  DelayLength=1
  Detect Rise Positive : simulink/Logic and Bit Operations/Detect Rise Positive  vinit=0  OutDataTypeStr=boolean
  Discrete-Time Integrator : DiscreteIntegrator  IntegratorMethod=Accumulation: Forward Euler  gainval=1  ExternalReset=level  SampleTime=-1  LimitOutput=on  UpperSaturationLimit=1e6  LowerSaturationLimit=0  ICPrevOutput=DiscIntNeverNeededParam  ICPrevScaledInput=DiscIntNeverNeededParam
  Logical Operator : Logic  Operator=NOT  AllPortsSameDT=off  OutDataTypeStr=boolean
  Logical Operator1 : Logic  Operator=OR  AllPortsSameDT=off  OutDataTypeStr=boolean
  Multiply : Product
  y : Outport
  wires:
  Multiply/1 -> y/1
  Delay/1 -> Multiply/2, Logical Operator1/2
  Logical Operator1/1 -> Delay/1
  Detect Rise Positive/1 -> Logical Operator1/1
  Compare To Constant2/1 -> Detect Rise Positive/1
  u/1 -> Compare To Constant1/1, Compare To Constant2/1
  Compare To Constant1/1 -> Discrete-Time Integrator/2
  Constant/1 -> Discrete-Time Integrator/1
  Compare To Constant/1 -> Logical Operator/1
  Logical Operator/1 -> Multiply/1
  Discrete-Time Integrator/1 -> Compare To Constant/1

== system INS/Data_Fusion/Translation_Filter/TF_Data_PreProcess/Transfer_Filter_Control/Sensor_Valid/Horizon_Sensor_Valid/valid_hold1 ==
  u : Inport
  Compare To Constant : simulink/Logic and Bit Operations/Compare To Constant  relop=>=  const=time_out  OutDataTypeStr=boolean
  Compare To Constant1 : simulink/Logic and Bit Operations/Compare To Constant  relop=>  const=0  OutDataTypeStr=boolean
  Compare To Constant2 : simulink/Logic and Bit Operations/Compare To Constant  relop=>  const=0  OutDataTypeStr=boolean
  Constant : Constant  Value=INS_EXPORT.period  OutDataTypeStr=Inherit: Inherit via back propagation
  Delay : Delay  DelayLength=1
  Detect Rise Positive : simulink/Logic and Bit Operations/Detect Rise Positive  vinit=0  OutDataTypeStr=boolean
  Discrete-Time Integrator : DiscreteIntegrator  IntegratorMethod=Accumulation: Forward Euler  gainval=1  ExternalReset=level  SampleTime=-1  LimitOutput=on  UpperSaturationLimit=1e6  LowerSaturationLimit=0  ICPrevOutput=DiscIntNeverNeededParam  ICPrevScaledInput=DiscIntNeverNeededParam
  Logical Operator : Logic  Operator=NOT  AllPortsSameDT=off  OutDataTypeStr=boolean
  Logical Operator1 : Logic  Operator=OR  AllPortsSameDT=off  OutDataTypeStr=boolean
  Multiply : Product
  y : Outport
  wires:
  Discrete-Time Integrator/1 -> Compare To Constant/1
  Logical Operator/1 -> Multiply/1
  Compare To Constant/1 -> Logical Operator/1
  Constant/1 -> Discrete-Time Integrator/1
  Compare To Constant1/1 -> Discrete-Time Integrator/2
  u/1 -> Compare To Constant2/1, Compare To Constant1/1
  Compare To Constant2/1 -> Detect Rise Positive/1
  Detect Rise Positive/1 -> Logical Operator1/1
  Logical Operator1/1 -> Delay/1
  Delay/1 -> Logical Operator1/2, Multiply/2
  Multiply/1 -> y/1

== system INS/Data_Fusion/Translation_Filter/TF_Data_PreProcess/Transfer_Filter_Control/Sensor_Valid/Vertical_Sensor_Valid/valid_hold ==
  u : Inport
  Compare To Constant : simulink/Logic and Bit Operations/Compare To Constant  relop=>=  const=time_out  OutDataTypeStr=boolean
  Compare To Constant1 : simulink/Logic and Bit Operations/Compare To Constant  relop=>  const=0  OutDataTypeStr=boolean
  Compare To Constant2 : simulink/Logic and Bit Operations/Compare To Constant  relop=>  const=0  OutDataTypeStr=boolean
  Constant : Constant  Value=INS_EXPORT.period  OutDataTypeStr=Inherit: Inherit via back propagation
  Delay : Delay  DelayLength=1
  Detect Rise Positive : simulink/Logic and Bit Operations/Detect Rise Positive  vinit=0  OutDataTypeStr=boolean
  Discrete-Time Integrator : DiscreteIntegrator  IntegratorMethod=Accumulation: Forward Euler  gainval=1  ExternalReset=level  SampleTime=-1  LimitOutput=on  UpperSaturationLimit=1e6  LowerSaturationLimit=0  ICPrevOutput=DiscIntNeverNeededParam  ICPrevScaledInput=DiscIntNeverNeededParam
  Logical Operator : Logic  Operator=NOT  AllPortsSameDT=off  OutDataTypeStr=boolean
  Logical Operator1 : Logic  Operator=OR  AllPortsSameDT=off  OutDataTypeStr=boolean
  Multiply : Product
  y : Outport
  wires:
  Multiply/1 -> y/1
  Delay/1 -> Multiply/2, Logical Operator1/2
  Logical Operator1/1 -> Delay/1
  Detect Rise Positive/1 -> Logical Operator1/1
  Compare To Constant2/1 -> Detect Rise Positive/1
  u/1 -> Compare To Constant1/1, Compare To Constant2/1
  Compare To Constant1/1 -> Discrete-Time Integrator/2
  Constant/1 -> Discrete-Time Integrator/1
  Compare To Constant/1 -> Logical Operator/1
  Logical Operator/1 -> Multiply/1
  Discrete-Time Integrator/1 -> Compare To Constant/1

== system INS/Data_Fusion/Translation_Filter/TF_Data_PreProcess/Transfer_Filter_Control/Sensor_Valid/Vertical_Sensor_Valid/valid_hold1 ==
  u : Inport
  Compare To Constant : simulink/Logic and Bit Operations/Compare To Constant  relop=>=  const=time_out  OutDataTypeStr=boolean
  Compare To Constant1 : simulink/Logic and Bit Operations/Compare To Constant  relop=>  const=0  OutDataTypeStr=boolean
  Compare To Constant2 : simulink/Logic and Bit Operations/Compare To Constant  relop=>  const=0  OutDataTypeStr=boolean
  Constant : Constant  Value=INS_EXPORT.period  OutDataTypeStr=Inherit: Inherit via back propagation
  Delay : Delay  DelayLength=1
  Detect Rise Positive : simulink/Logic and Bit Operations/Detect Rise Positive  vinit=0  OutDataTypeStr=boolean
  Discrete-Time Integrator : DiscreteIntegrator  IntegratorMethod=Accumulation: Forward Euler  gainval=1  ExternalReset=level  SampleTime=-1  LimitOutput=on  UpperSaturationLimit=1e6  LowerSaturationLimit=0  ICPrevOutput=DiscIntNeverNeededParam  ICPrevScaledInput=DiscIntNeverNeededParam
  Logical Operator : Logic  Operator=NOT  AllPortsSameDT=off  OutDataTypeStr=boolean
  Logical Operator1 : Logic  Operator=OR  AllPortsSameDT=off  OutDataTypeStr=boolean
  Multiply : Product
  y : Outport
  wires:
  Discrete-Time Integrator/1 -> Compare To Constant/1
  Logical Operator/1 -> Multiply/1
  Compare To Constant/1 -> Logical Operator/1
  Constant/1 -> Discrete-Time Integrator/1
  Compare To Constant1/1 -> Discrete-Time Integrator/2
  u/1 -> Compare To Constant2/1, Compare To Constant1/1
  Compare To Constant2/1 -> Detect Rise Positive/1
  Detect Rise Positive/1 -> Logical Operator1/1
  Logical Operator1/1 -> Delay/1
  Delay/1 -> Logical Operator1/2, Multiply/2
  Multiply/1 -> y/1

== system INS/Data_Fusion/Rotation_Filter/AHRS/Correct/Attitude_Correction/Attitude_Correct/Acc_Correct/Heading_Correct ==
  acc_est_O_mPs2 : Inport
  acc_meas_O_mPs2 : Inport  Port=2
  acc_meas_valid : Inport  Port=3
  Cross Product : FMT_Model_Lib/Math/Cross Product
      settings: SourceProductName=FMT Toolbox
  Dead Zone2 : DeadZone  LowerValue=-0.2  UpperValue=0.2  SaturateOnIntegerOverflow=on
  Demux : Demux  Outputs=3
  Demux1 : Demux  Outputs=3
  Gain : Gain  Gain=INS_PARAM.HEADING_CORR_GAIN  OutDataTypeStr=single
  Gain1 : Gain  Gain=0
  Gain2 : Gain  Gain=0
  Multiply : Product
  Mux1 : Mux  Inputs=3
  Mux2 : Mux  Inputs=3
  Saturation : Saturate
  heading_correct : Outport
  wires:
  Dead Zone2/1 -> Gain/1
  Saturation/1 -> Multiply/1
  Mux1/1 -> Cross Product/2
  Cross Product/1 -> Dead Zone2/1
  Demux/1 -> Mux1/1
  acc_meas_valid/1 -> Multiply/2
  Multiply/1 -> heading_correct/1
  Gain/1 -> Saturation/1
  acc_meas_O_mPs2/1 -> Demux/1
  Demux/2 -> Mux1/2
  Demux/3 -> Gain1/1
  Gain1/1 -> Mux1/3
  Demux1/2 -> Mux2/2
  Mux2/1 -> Cross Product/1
  Gain2/1 -> Mux2/3
  Demux1/1 -> Mux2/1
  Demux1/3 -> Gain2/1
  acc_est_O_mPs2/1 -> Demux1/1

== system INS/Data_Fusion/Rotation_Filter/AHRS/Correct/Attitude_Correction/Attitude_Correct/Acc_Correct/Verticle_Correct ==
  acc_est_O_mPs2 : Inport
  acc_meas_O_mPs2 : Inport  Port=2
  Cross Product : FMT_Model_Lib/Math/Cross Product
      settings: SourceProductName=FMT Toolbox
  Gain : Gain  Gain=[INS_PARAM.ATT_CORR_GAIN;INS_PARAM.ATT_CORR_GAIN;0]
  Saturation : Subsystem
  Vector Normalize : FMT_Model_Lib/Math/Vector Normalize
      settings: SourceProductName=FMT Toolbox
  Vector Normalize1 : FMT_Model_Lib/Math/Vector Normalize
      settings: SourceProductName=FMT Toolbox
  vert_correct : Outport
  wires:
  Saturation/1(y) -> Gain/1
  Cross Product/1 -> Saturation/1(u)
  Vector Normalize/1 -> Cross Product/1
  acc_meas_O_mPs2/1 -> Vector Normalize1/1
  Gain/1 -> vert_correct/1
  acc_est_O_mPs2/1 -> Vector Normalize/1
  Vector Normalize1/1 -> Cross Product/2

== system INS/Data_Fusion/Rotation_Filter/AHRS/Correct/Attitude_Correction/Attitude_Correct/Acc_Estimator/Estimate_Acc ==
  gps_meas_valid : Inport
  Sensor_Data : Inport  Port=2
  Rotation_Data : Inport  Port=3
  Bus Selector : BusSelector  OutputSignals=IMU_Data.acc_B_mPs2
  Bus Selector1 : BusSelector  OutputSignals=M_OB
  Delay : Delay  DelayLengthSource=Input port  DelayLengthUpperLimit=200
      settings: InputPortMap=u0,p1
  GPS_Delay : Constant  Value=200/INS_EXPORT.period  OutDataTypeStr=uint16
  Multiply : Product  Multiplication=Matrix(*)
  Multiply2 : Product  OutDataTypeStr=single
  Second Order LPF : FMT_Model_Lib/Filter/Second Order LPF  fc=10  zeta=0.707
      settings: SourceProductName=FMT Toolbox
  acc_est_O_mPs2 : Outport
  wires:
  Second Order LPF/1 -> Delay/1
  Multiply/1 -> Second Order LPF/1  "acc_O"
  Bus Selector/1 -> Multiply/2  "<acc_B_mPs2>"
  Bus Selector1/1 -> Multiply/1  "<M_OB>"
  Rotation_Data/1 -> Bus Selector1/1
  Sensor_Data/1 -> Bus Selector/1
  Delay/1 -> acc_est_O_mPs2/1
  Multiply2/1 -> Delay/2
  GPS_Delay/1 -> Multiply2/2
  gps_meas_valid/1 -> Multiply2/1

== system INS/Data_Fusion/Rotation_Filter/AHRS/Correct/Attitude_Correction/Attitude_Correct/Acc_Estimator/Measure_Acc ==
  Sensor_Data : Inport
  Bus_Selection : Subsystem
  Detect Increase : simulink/Logic and Bit Operations/Detect Increase  vinit=0.0  OutDataTypeStr=boolean
  GPS_Meas_Acc : Subsystem  mask{fc=10, zeta=1}
      mask prompts: fc "Cut-off frequency (Hz)"; zeta "Damping factor"
  Valid_Check : Subsystem
  gps_meas_valid : Outport
  gps_meas_acc : Outport  Port=2
  wires:
  Valid_Check/1(gps_meas_acc_valid) -> gps_meas_valid/1, GPS_Meas_Acc/Enable, Detect Increase/1
  Detect Increase/1 -> GPS_Meas_Acc/1(reset)
  GPS_Meas_Acc/1(gps_acc_O_mPs2) -> gps_meas_acc/1
  Bus_Selection/1(gps_vel_O_mPs) -> GPS_Meas_Acc/2(gps_vel_O_mPs)
  Sensor_Data/1 -> Bus_Selection/1(Sensor_Data), Valid_Check/1(Sensor_Data)

== system INS/Data_Fusion/Translation_Filter/CF/Bus_Constructor/Bus_Select/WGS84_Position/WGS84_Position/safe_divide ==
  u1 : Inport
  u2 : Inport  Port=2
  Divide : Product  Inputs=*/
  Zero_Value_Exclusion : Subsystem
  y : Outport
  wires:
  Zero_Value_Exclusion/1(y) -> Divide/2
  Divide/1 -> y/1
  u1/1 -> Divide/1
  u2/1 -> Zero_Value_Exclusion/1(u)

== system INS/Data_Fusion/Translation_Filter/CF/Horizontal_Filter/Correct/GPS_Correct/Measurement/Bias_Estimation ==
  TF_Data : Inport
  X : Inport  Port=2
  xy_meas_m : Inport  Port=3
  Bias : Subsystem
  Sum1 : Sum  Inputs=|++
  bias_update : Outport
  xy_O_m : Outport  Port=2
  wires:
  TF_Data/1 -> Bias/3(TF_Data)
  X/1 -> Bias/2(X)
  Sum1/1 -> xy_O_m/1
  Bias/1(bias) -> Sum1/2
  xy_meas_m/1 -> Sum1/1, Bias/1(xy_meas_m)  "gps_xy_m"
  Bias/2(bias_update) -> bias_update/1

== system INS/Data_Fusion/Translation_Filter/CF/Horizontal_Filter/Predict/Propagate/States_Init/Pos_Init ==
  TF_Data : Inport
  Bus Selector : BusSelector  OutputSignals=Sensor_Status.GPS_Status.gps_vaid
  GPS_Pos_Init : Subsystem
  XY_0 : Outport
  wires:
  TF_Data/1 -> GPS_Pos_Init/1(TF_Data), Bus Selector/1
  GPS_Pos_Init/1(X_0) -> XY_0/1  "xy_0"
  Bus Selector/1 -> GPS_Pos_Init/Enable  "<gps_vaid>"

== system INS/Data_Fusion/Translation_Filter/CF/Horizontal_Filter/Predict/Propagate/States_Init/Vel_Init ==
  TF_Data : Inport
  Bus Selector : BusSelector  OutputSignals=Sensor_Status.GPS_Status.gps_vaid
  GPS_Vel_Init : Subsystem
  vel_NE_0 : Outport
  wires:
  TF_Data/1 -> GPS_Vel_Init/1(Processed_Data), Bus Selector/1
  GPS_Vel_Init/1(Vel_NE_0) -> vel_NE_0/1  "vel_NE_0"
  Bus Selector/1 -> GPS_Vel_Init/Enable  "<gps_vaid>"

== system INS/Data_Fusion/Translation_Filter/CF/Verticle_Filter/Correct/Baro_Correct/Baro_Correct/Error_Hold ==
  in : Inport
  update : Inport  Port=2
  Delay : Delay  DelayLength=1
  Gain : Gain  Gain=INS_CONST.dt  OutDataTypeStr=Inherit: Same as input
  Switch : Switch  Criteria=u2 > Threshold
  out : Outport
  wires:
  update/1 -> Switch/2
  Switch/1 -> Delay/1, Gain/1
  in/1 -> Switch/1
  Delay/1 -> Switch/3
  Gain/1 -> out/1

== system INS/Data_Fusion/Translation_Filter/CF/Verticle_Filter/Correct/Baro_Correct/Baro_Correct/Error_Scaling ==
  errror_in : Inport
  Gain : Gain  Gain=INS_PARAM.BARO_BIAS_AZ_CORR_GAIN
  Gain1 : Gain  Gain=-INS_PARAM.BARO_VZ_CORR_GAIN
  Gain2 : Gain  Gain=INS_PARAM.BARO_H_CORR_GAIN
  Mux : Mux  Inputs=3
  Saturation : Saturate  UpperLimit=1  LowerLimit=-1
  errror_out : Outport
  wires:
  errror_in/1 -> Saturation/1
  Gain2/1 -> Mux/1
  Gain1/1 -> Mux/2
  Gain/1 -> Mux/3
  Mux/1 -> errror_out/1
  Saturation/1 -> Gain/1, Gain2/1, Gain1/1

== system INS/Data_Fusion/Translation_Filter/CF/Verticle_Filter/Correct/Baro_Correct/Baro_Correct/Estimate_States ==
  note: Delay compensate due to sensor
      | measurement delay
  X : Inport
  reset : Inport  Port=2
  Selector : Selector  InputPortWidth=3  IndexOptions=Index vector (dialog)  Indices=[1]  OutputSizes=1
  x_delay : Delay  DelayLength=INS_PARAM.BARO_H_DELAY/INS_EXPORT_VALUE.period  InitialConditionSource=Input port  ExternalReset=Rising
      settings: InputPortMap=u0,r5,p4
  HX : Outport
  wires:
  reset/1 -> x_delay/2
  Selector/1 -> x_delay/1, x_delay/3  "HX"
  X/1 -> Selector/1
  x_delay/1 -> HX/1

== system INS/Data_Fusion/Translation_Filter/CF/Verticle_Filter/Correct/Baro_Correct/Baro_Correct/Measurement ==
  X : Inport
  TF_Data : Inport  Port=2
  Bias_Estimation : Subsystem
  Bus Selector : BusSelector  OutputSignals=Sensor_Meas.Baro_Meas.h_R_m
  Sum1 : Sum  Inputs=|++
  Z : Outport
  bias_update : Outport  Port=2
  wires:
  Bus Selector/1 -> Bias_Estimation/1(h_m), Sum1/1  "<h_R_m>"
  Bias_Estimation/1(bias) -> Sum1/2
  X/1 -> Bias_Estimation/3(X)
  TF_Data/1 -> Bias_Estimation/2(TF_Data), Bus Selector/1
  Sum1/1 -> Z/1
  Bias_Estimation/2(bias_update) -> bias_update/1

== system INS/Data_Fusion/Translation_Filter/CF/Verticle_Filter/Correct/GPS_Correct/GPS_Correct/Error_Hold ==
  in : Inport
  update : Inport  Port=2
  Gain3 : Gain  Gain=INS_CONST.dt  OutDataTypeStr=Inherit: Same as input
  Memory : Memory
  Switch : Switch  Criteria=u2 > Threshold
  out : Outport
  wires:
  update/1 -> Switch/2
  Switch/1 -> Memory/1, Gain3/1
  in/1 -> Switch/1
  Memory/1 -> Switch/3
  Gain3/1 -> out/1

== system INS/Data_Fusion/Translation_Filter/CF/Verticle_Filter/Correct/GPS_Correct/GPS_Correct/Error_Scaling ==
  error_in : Inport
  Demux : Demux  Outputs=2
  Gain : Gain  Gain=INS_PARAM.GPS_VEL_CORR_GAIN  OutDataTypeStr=single
  Gain1 : Gain  Gain=INS_PARAM.GPS_POS_CORR_GAIN  OutDataTypeStr=single
  Gain2 : Gain  Gain=-INS_PARAM.GPS_BIAS_A_CORR_GAIN  OutDataTypeStr=single
  Gain3 : Gain  Commented=on  Gain=1.5  OutDataTypeStr=single
  Mux : Mux  Inputs=3
  error_out : Outport
  wires:
  error_in/1 -> Demux/1
  Demux/1 -> Gain1/1
  Demux/2 -> Gain2/1, Gain/1
  Gain2/1 -> Mux/3
  Mux/1 -> error_out/1
  Gain1/1 -> Mux/1
  Gain/1 -> Mux/2

== system INS/Data_Fusion/Translation_Filter/CF/Verticle_Filter/Correct/GPS_Correct/GPS_Correct/Estimate_State ==
  X : Inport
  reset : Inport  Port=2
  Mux : Mux  Inputs=2
  Reshape : Reshape  OutputDimensionality=Customize  OutputDimensions=[2,1]
  Selector : Selector  InputPortWidth=3  IndexOptions=Index vector (dialog)  Indices=[1]  OutputSizes=1
  Selector1 : Selector  InputPortWidth=3  IndexOptions=Index vector (dialog)  Indices=[2]  OutputSizes=1
  h_delay : Delay  DelayLength=INS_PARAM.GPS_POS_DELAY/INS_EXPORT.period  InitialConditionSource=Input port  ExternalReset=Rising
      settings: InputPortMap=u0,r5,p4
  vd_delay : Delay  DelayLength=INS_PARAM.GPS_VEL_DELAY/INS_EXPORT.period  InitialConditionSource=Input port  ExternalReset=Rising
      settings: InputPortMap=u0,r5,p4
  HX : Outport
  wires:
  reset/1 -> h_delay/2, vd_delay/2
  h_delay/1 -> Mux/1
  vd_delay/1 -> Mux/2
  Reshape/1 -> HX/1
  Mux/1 -> Reshape/1
  Selector/1 -> h_delay/3, h_delay/1
  X/1 -> Selector1/1, Selector/1
  Selector1/1 -> vd_delay/3, vd_delay/1

== system INS/Data_Fusion/Translation_Filter/CF/Verticle_Filter/Correct/GPS_Correct/GPS_Correct/Measurement ==
  X : Inport
  TF_Data : Inport  Port=2
  Bias_Estimation : Subsystem
  Bus Selector : BusSelector  OutputSignals=Sensor_Meas.GPS_Meas.h_m,TF_Control.WGS84_Ref.WGS84_pos_ref.h_0_m
  Bus Selector1 : BusSelector  OutputSignals=Sensor_Meas.GPS_Meas.vd_mPs
  Data Type Conversion : DataTypeConversion  OutDataTypeStr=single
  Mux : Mux  Inputs=2
  Sum : Sum  Inputs=|+-
  Sum1 : Sum  Inputs=|++
  Z : Outport
  bias_update : Outport  Port=2
  wires:
  Data Type Conversion/1 -> Sum1/1, Bias_Estimation/1(h_m)
  Bus Selector/2 -> Sum/2  "<h_0_m>"
  Bus Selector/1 -> Sum/1  "<h_m>"
  TF_Data/1 -> Bias_Estimation/3(TF_Data), Bus Selector1/1, Bus Selector/1
  Sum/1 -> Data Type Conversion/1
  X/1 -> Bias_Estimation/2(X)
  Sum1/1 -> Mux/1
  Bias_Estimation/1(bias) -> Sum1/2
  Bias_Estimation/2(bias_update) -> bias_update/1
  Bus Selector1/1 -> Mux/2  "<vd_mPs>"
  Mux/1 -> Z/1

== system INS/Data_Fusion/Translation_Filter/CF/Verticle_Filter/Predict/Propagate/States_Init/Baro_Height_Init ==
  TF_Data : Inport
  Bus Selector : BusSelector  OutputSignals=Sensor_Enable.vert_select.baro_enable
  Reference_Height : Subsystem
  h_0 : Outport
  vel_D : Outport  Port=2
  wires:
  TF_Data/1 -> Bus Selector/1, Reference_Height/1(TF_Data)
  Reference_Height/1(h_R_m) -> h_0/1
  Bus Selector/1 -> Reference_Height/Enable  "<baro_enable>"
  Reference_Height/2(vel_D_mPs) -> vel_D/1

== system INS/Data_Fusion/Translation_Filter/CF/Verticle_Filter/Predict/Propagate/States_Init/GPS_Height_Init ==
  TF_Data : Inport
  Bus Selector : BusSelector  OutputSignals=Sensor_Enable.vert_select.gps_enable
  Reference_Height : Subsystem
  h_0 : Outport
  vel_D : Outport  Port=2
  wires:
  TF_Data/1 -> Bus Selector/1, Reference_Height/1(TF_Data)
  Reference_Height/1(h_R_m) -> h_0/1
  Bus Selector/1 -> Reference_Height/Enable  "<gps_enable>"
  Reference_Height/2(vel_D_mPs) -> vel_D/1

== system INS/Data_Fusion/Rotation_Filter/AHRS/Correct/Attitude_Correction/Attitude_Correct/Acc_Correct/Verticle_Correct/Saturation ==
  u : Inport
  Constant1 : Constant  Value=1e-4  OutDataTypeStr=Inherit: Inherit via back propagation
  Divide : Product  Inputs=**/
  Divide1 : Product  Inputs=*/
  Divide2 : Product  Inputs=**
  MinMax : MinMax  Function=max  Inputs=2
  Saturation : Saturate  UpperLimit=pi/2  LowerLimit=-pi/2
  Trigonometric Function : Trigonometry
  Vector Modulus : FMT_Model_Lib/Math/Vector Modulus
      settings: SourceProductName=FMT Toolbox
  max : Constant  Value=10/180*pi  OutDataTypeStr=single
  y : Outport
  wires:
  Constant1/1 -> MinMax/2
  Saturation/1 -> Trigonometric Function/1
  u/1 -> Vector Modulus/1, Divide/1
  Trigonometric Function/1 -> Divide2/1
  Divide/1 -> y/1
  Vector Modulus/1 -> Divide1/1, MinMax/1
  Divide1/1 -> Saturation/1
  Divide2/1 -> Divide/2
  max/1 -> Divide1/2, Divide2/2
  MinMax/1 -> Divide/3

== system INS/Data_Fusion/Rotation_Filter/AHRS/Correct/Attitude_Correction/Attitude_Correct/Acc_Estimator/Measure_Acc/Bus_Selection ==
  Sensor_Data : Inport
  Bus Selector2 : BusSelector  OutputSignals=GPS_Data.vn_mPs,GPS_Data.ve_mPs,GPS_Data.vd_mPs
  Mux : Mux  Inputs=3
  gps_vel_O_mPs : Outport
  wires:
  Sensor_Data/1 -> Bus Selector2/1
  Bus Selector2/1 -> Mux/1  "<vn_mPs>"
  Bus Selector2/2 -> Mux/2  "<ve_mPs>"
  Bus Selector2/3 -> Mux/3  "<vd_mPs>"
  Mux/1 -> gps_vel_O_mPs/1
